simulink model "deadbeat_running_control"  (R2016b)
settings: configuration reference "Configuration1khz" (kept outside this file)
undefined symbols (not defined in the file or in its folder): A_kalman_no_position, A_kalman_transverse, A_kalman_vertical, A_lpf_accelerometer, A_lpf_contact, A_lpf_imu, A_lpf_lateral_angle, B1_lpf_accelerometer, B1_lpf_contact, B1_lpf_imu, B1_lpf_lateral_angle, B2_lpf_accelerometer, B2_lpf_contact, B2_lpf_imu, B2_lpf_lateral_angle, B_dx_versus_x0, B_kalman_no_position, B_kalman_transverse, B_kalman_vertical, backwards_K_sag_of_t, backwards_P_sag_of_t, C_kalman_no_position, C_kalman_transverse, C_kalman_vertical, com_leg_motor, com_torso, contact_threshold, d_ankle_to_foot, d_vertical_com, desired_com_forward_velocity, desired_com_lateral_velocity, desired_standing_torso_pitch, desired_standing_torso_roll, desired_standing_z, desired_torso_pitch, desired_torso_roll, DiscIntNeverNeededParam, Discrete, enable_bouncing, fdesignblkfcn, flight_duration, forward_dx_of_dxstar, forward_x_of_dxstar, g, gcbh, HIP_MTR_MAX_CONT_TORQUE, HIP_MTR_MAX_TORQUE, i_leg_motor, i_robot, i_torso, initial_dx_estimate, initial_dx_takeoff_history, initial_dx_touchdown_history, initial_dy_estimate, initial_dy_takeoff_history, initial_dy_touchdown_history, initial_dz_estimate, initial_leg_selection, initial_target_dx_history, initial_target_dy_history ... (+80)
libraries: simulink x22, ctrlSharedLib x4, dsparch4 x2
(part 3 of 7)

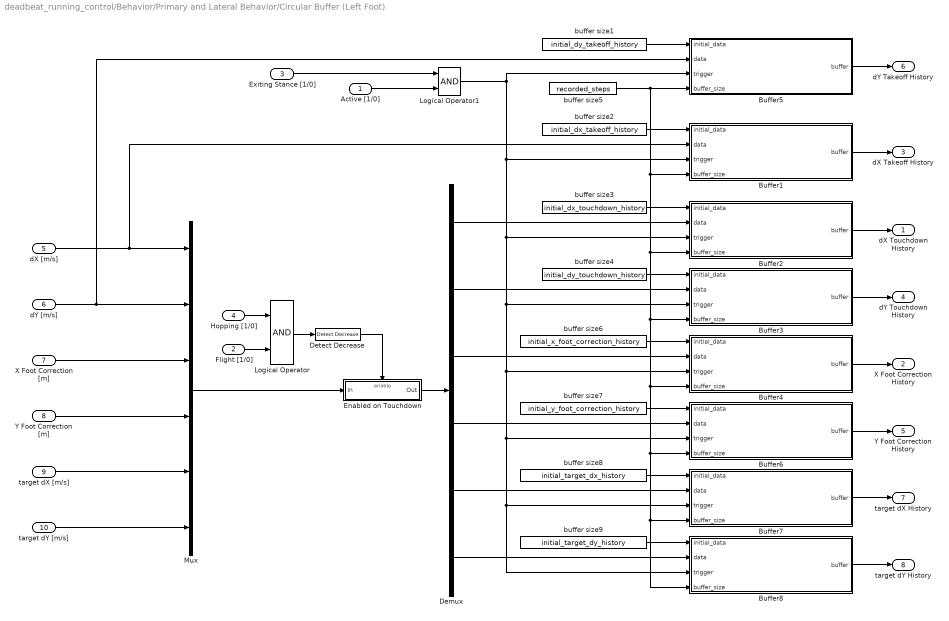
== system deadbeat_running_control/Behavior/Primary and Lateral Behavior/Circular Buffer (Left Foot) ==
  Active [1/0] : Inport
  Flight [1/0] : Inport  Port=2
  Exiting Stance [1/0] : Inport  Port=3
  Hopping [1/0] : Inport  Port=4
  dX [m/s] : Inport  Port=5
  dY [m/s] : Inport  Port=6
  X Foot Correction [m] : Inport  Port=7
  Y Foot Correction [m] : Inport  Port=8
  target dX [m/s] : Inport  Port=9
  target dY [m/s] : Inport  Port=10
  Buffer1 : MATLAB Function  TreatAsAtomicUnit=on  SystemSampleTime=sample_time
  Buffer2 : MATLAB Function  TreatAsAtomicUnit=on  SystemSampleTime=sample_time
  Buffer3 : MATLAB Function  TreatAsAtomicUnit=on  SystemSampleTime=sample_time
  Buffer4 : MATLAB Function  TreatAsAtomicUnit=on  SystemSampleTime=sample_time
  Buffer5 : MATLAB Function  TreatAsAtomicUnit=on  SystemSampleTime=sample_time
  Buffer6 : MATLAB Function  TreatAsAtomicUnit=on  SystemSampleTime=sample_time
  Buffer7 : MATLAB Function  TreatAsAtomicUnit=on  SystemSampleTime=sample_time
  Buffer8 : MATLAB Function  TreatAsAtomicUnit=on  SystemSampleTime=sample_time
  Demux : Demux  Outputs=6
  Detect Decrease : simulink/Logic and Bit Operations/Detect Decrease  vinit=0.0  InputProcessing=Inherited  OutDataTypeStr=boolean
  Enabled on Touchdown : Subsystem  TreatAsAtomicUnit=on
  Logical Operator : Logic  AllPortsSameDT=off  OutDataTypeStr=boolean
  Logical Operator1 : Logic  AllPortsSameDT=off  OutDataTypeStr=boolean
  Mux : Mux  Inputs=6
  buffer size1 : Constant  Value=initial_dy_takeoff_history
  buffer size2 : Constant  Value=initial_dx_takeoff_history
  buffer size3 : Constant  Value=initial_dx_touchdown_history
  buffer size4 : Constant  Value=initial_dy_touchdown_history
  buffer size5 : Constant  Value=recorded_steps
  buffer size6 : Constant  Value=initial_x_foot_correction_history
  buffer size7 : Constant  Value=initial_y_foot_correction_history
  buffer size8 : Constant  Value=initial_target_dx_history
  buffer size9 : Constant  Value=initial_target_dy_history
  "dX Touchdown History " : Outport
  X Foot Correction History : Outport  Port=2
  dX Takeoff History : Outport  Port=3
  "dY Touchdown History " : Outport  Port=4
  Y Foot Correction History : Outport  Port=5
  dY Takeoff History : Outport  Port=6
  target dX History : Outport  Port=7
  target dY History : Outport  Port=8
  wires:
  Enabled on Touchdown/1(Out) -> Demux/1
  Mux/1 -> Enabled on Touchdown/1(In)
  Logical Operator/1 -> Detect Decrease/1
  Flight [1/0]/1 -> Logical Operator/2
  dX [m/s]/1 -> Mux/1, Buffer1/2(data)
  dY [m/s]/1 -> Mux/2, Buffer5/2(data)
  Hopping [1/0]/1 -> Logical Operator/1
  Logical Operator1/1 -> Buffer7/3(trigger), Buffer8/3(trigger), Buffer6/3(trigger), Buffer4/3(trigger), Buffer3/3(trigger), Buffer2/3(trigger), Buffer1/3(trigger), Buffer5/3(trigger)
  target dY [m/s]/1 -> Mux/6
  Demux/5 -> Buffer7/2(data)
  Demux/6 -> Buffer8/2(data)
  buffer size5/1 -> Buffer5/4(buffer_size), Buffer7/4(buffer_size), Buffer8/4(buffer_size), Buffer6/4(buffer_size), Buffer4/4(buffer_size), Buffer3/4(buffer_size), Buffer2/4(buffer_size), Buffer1/4(buffer_size)
  Buffer8/1(buffer) -> target dY History/1
  Buffer7/1(buffer) -> target dX History/1
  target dX [m/s]/1 -> Mux/5
  Demux/4 -> Buffer6/2(data)
  Y Foot Correction [m]/1 -> Mux/4
  Buffer5/1(buffer) -> dY Takeoff History/1
  Demux/2 -> Buffer3/2(data)
  Buffer6/1(buffer) -> Y Foot Correction History/1
  Buffer3/1(buffer) -> "dY Touchdown History "/1
  X Foot Correction [m]/1 -> Mux/3
  Demux/3 -> Buffer4/2(data)
  Demux/1 -> Buffer2/2(data)
  Buffer1/1(buffer) -> dX Takeoff History/1
  Buffer4/1(buffer) -> X Foot Correction History/1
  Detect Decrease/1 -> Enabled on Touchdown/Enable
  Buffer2/1(buffer) -> "dX Touchdown History "/1
  buffer size1/1 -> Buffer5/1(initial_data)
  buffer size2/1 -> Buffer1/1(initial_data)
  buffer size3/1 -> Buffer2/1(initial_data)
  buffer size4/1 -> Buffer3/1(initial_data)
  buffer size6/1 -> Buffer4/1(initial_data)
  buffer size7/1 -> Buffer6/1(initial_data)
  buffer size8/1 -> Buffer7/1(initial_data)
  buffer size9/1 -> Buffer8/1(initial_data)
  Active [1/0]/1 -> Logical Operator1/2
  Exiting Stance [1/0]/1 -> Logical Operator1/1

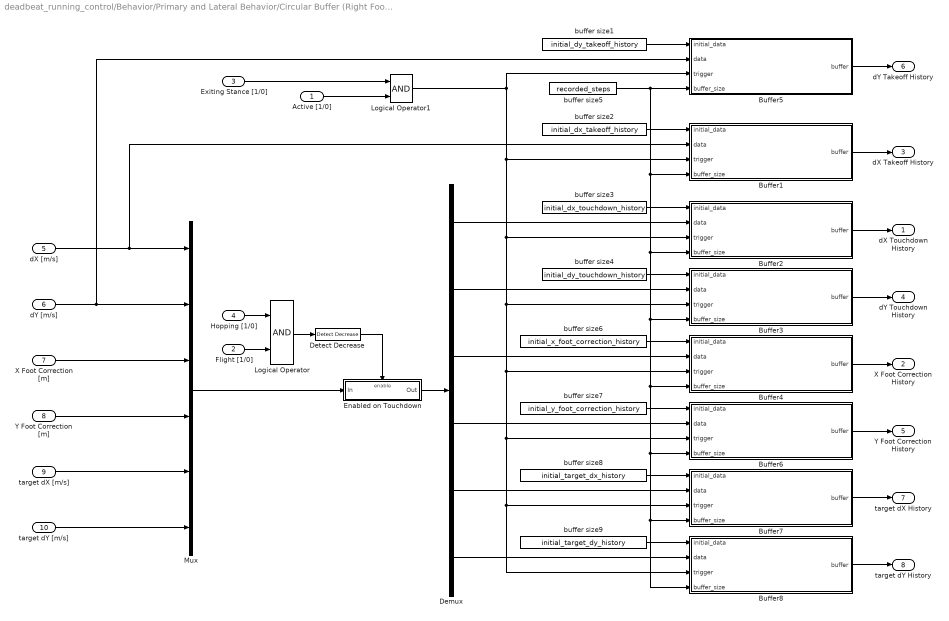
== system deadbeat_running_control/Behavior/Primary and Lateral Behavior/Circular Buffer (Right Foot) ==
  Active [1/0] : Inport
  Flight [1/0] : Inport  Port=2
  Exiting Stance [1/0] : Inport  Port=3
  Hopping [1/0] : Inport  Port=4
  dX [m/s] : Inport  Port=5
  dY [m/s] : Inport  Port=6
  X Foot Correction [m] : Inport  Port=7
  Y Foot Correction [m] : Inport  Port=8
  target dX [m/s] : Inport  Port=9
  target dY [m/s] : Inport  Port=10
  Buffer1 : MATLAB Function  TreatAsAtomicUnit=on  SystemSampleTime=sample_time
  Buffer2 : MATLAB Function  TreatAsAtomicUnit=on  SystemSampleTime=sample_time
  Buffer3 : MATLAB Function  TreatAsAtomicUnit=on  SystemSampleTime=sample_time
  Buffer4 : MATLAB Function  TreatAsAtomicUnit=on  SystemSampleTime=sample_time
  Buffer5 : MATLAB Function  TreatAsAtomicUnit=on  SystemSampleTime=sample_time
  Buffer6 : MATLAB Function  TreatAsAtomicUnit=on  SystemSampleTime=sample_time
  Buffer7 : MATLAB Function  TreatAsAtomicUnit=on  SystemSampleTime=sample_time
  Buffer8 : MATLAB Function  TreatAsAtomicUnit=on  SystemSampleTime=sample_time
  Demux : Demux  Outputs=6
  Detect Decrease : simulink/Logic and Bit Operations/Detect Decrease  vinit=0.0  InputProcessing=Inherited  OutDataTypeStr=boolean
  Enabled on Touchdown : Subsystem  TreatAsAtomicUnit=on
  Logical Operator : Logic  AllPortsSameDT=off  OutDataTypeStr=boolean
  Logical Operator1 : Logic  AllPortsSameDT=off  OutDataTypeStr=boolean
  Mux : Mux  Inputs=6
  buffer size1 : Constant  Value=initial_dy_takeoff_history
  buffer size2 : Constant  Value=initial_dx_takeoff_history
  buffer size3 : Constant  Value=initial_dx_touchdown_history
  buffer size4 : Constant  Value=initial_dy_touchdown_history
  buffer size5 : Constant  Value=recorded_steps
  buffer size6 : Constant  Value=initial_x_foot_correction_history
  buffer size7 : Constant  Value=initial_y_foot_correction_history
  buffer size8 : Constant  Value=initial_target_dx_history
  buffer size9 : Constant  Value=initial_target_dy_history
  "dX Touchdown History " : Outport
  X Foot Correction History : Outport  Port=2
  dX Takeoff History : Outport  Port=3
  "dY Touchdown History " : Outport  Port=4
  Y Foot Correction History : Outport  Port=5
  dY Takeoff History : Outport  Port=6
  target dX History : Outport  Port=7
  target dY History : Outport  Port=8
  wires:
  buffer size9/1 -> Buffer8/1(initial_data)
  buffer size8/1 -> Buffer7/1(initial_data)
  buffer size7/1 -> Buffer6/1(initial_data)
  buffer size6/1 -> Buffer4/1(initial_data)
  buffer size4/1 -> Buffer3/1(initial_data)
  buffer size3/1 -> Buffer2/1(initial_data)
  buffer size2/1 -> Buffer1/1(initial_data)
  buffer size1/1 -> Buffer5/1(initial_data)
  Buffer2/1(buffer) -> "dX Touchdown History "/1
  Detect Decrease/1 -> Enabled on Touchdown/Enable
  Buffer4/1(buffer) -> X Foot Correction History/1
  Buffer1/1(buffer) -> dX Takeoff History/1
  Demux/1 -> Buffer2/2(data)
  Demux/3 -> Buffer4/2(data)
  X Foot Correction [m]/1 -> Mux/3
  Buffer3/1(buffer) -> "dY Touchdown History "/1
  Buffer6/1(buffer) -> Y Foot Correction History/1
  Demux/2 -> Buffer3/2(data)
  Buffer5/1(buffer) -> dY Takeoff History/1
  Y Foot Correction [m]/1 -> Mux/4
  Demux/4 -> Buffer6/2(data)
  target dX [m/s]/1 -> Mux/5
  Buffer7/1(buffer) -> target dX History/1
  Buffer8/1(buffer) -> target dY History/1
  buffer size5/1 -> Buffer1/4(buffer_size), Buffer2/4(buffer_size), Buffer3/4(buffer_size), Buffer4/4(buffer_size), Buffer6/4(buffer_size), Buffer8/4(buffer_size), Buffer7/4(buffer_size), Buffer5/4(buffer_size)
  Demux/6 -> Buffer8/2(data)
  Demux/5 -> Buffer7/2(data)
  target dY [m/s]/1 -> Mux/6
  Logical Operator1/1 -> Buffer5/3(trigger), Buffer1/3(trigger), Buffer2/3(trigger), Buffer3/3(trigger), Buffer4/3(trigger), Buffer6/3(trigger), Buffer8/3(trigger), Buffer7/3(trigger)
  Hopping [1/0]/1 -> Logical Operator/1
  dY [m/s]/1 -> Buffer5/2(data), Mux/2
  dX [m/s]/1 -> Buffer1/2(data), Mux/1
  Flight [1/0]/1 -> Logical Operator/2
  Logical Operator/1 -> Detect Decrease/1
  Mux/1 -> Enabled on Touchdown/1(In)
  Enabled on Touchdown/1(Out) -> Demux/1
  Exiting Stance [1/0]/1 -> Logical Operator1/1
  Active [1/0]/1 -> Logical Operator1/2

== system deadbeat_running_control/Behavior/Primary and Lateral Behavior/Closed Loop Compensation (Left Foot) ==
  dX Touchdown History : Inport
  X Foot Correction History : Inport  Port=2
  dX Takeoff History : Inport  Port=3
  dY Touchdown History : Inport  Port=4
  Y Foot Correction History : Inport  Port=5
  dY Takeoff History : Inport  Port=6
  target dX History : Inport  Port=7
  target dY History : Inport  Port=8
  dX [m/s] : Inport  Port=9
  dY [m/s] : Inport  Port=10
  target dX [m/s] : Inport  Port=11
  "target dY [m/s] " : Inport  Port=12
  "A, eps, c" : Scope  NumInputPorts=3
  A_x_no_bias : Gain
  A_y_no_bias : Gain
  CLOSED LOOP COMPENSATION X FOR VAIRABLE SPEED : MATLAB Function  TreatAsAtomicUnit=on
  CLOSED LOOP COMPENSATION Y FOR VAIRABLE SPEED : MATLAB Function  TreatAsAtomicUnit=on
  Constant4 : Constant  Value=B_dx_versus_x0
  ESTIMATE CLOSED LOOP ERROR X FOR VARIABLE SPEED : MATLAB Function  TreatAsAtomicUnit=on
  ESTIMATE CLOSED LOOP ERROR Y FOR VARIABLE SPEED : MATLAB Function  TreatAsAtomicUnit=on
  How much dx depends on x0 : Constant  Value=B_dx_versus_x0
  RealVsFakeWeight : Constant  Value=2
  RealVsFakeWeight1 : Constant  Value=2
  Sum : Sum  Inputs=|+-
  Sum1 : Sum  Inputs=|+-
  Terminator{2..7} (6 alike) : Terminator
  XY Foot Correction : Scope  NumInputPorts=2
  c_x_no_bias : Gain
  c_y_no_bias : Gain
  epsilon_x_no_bias : Gain
  epsilon_y_no_bias : Gain
  X Foot Correction [m] : Outport
  Y Foot Correction [m] : Outport  Port=2
  wires:
  RealVsFakeWeight1/1 -> ESTIMATE CLOSED LOOP ERROR Y FOR VARIABLE SPEED/5(W_real)
  Constant4/1 -> CLOSED LOOP COMPENSATION Y FOR VAIRABLE SPEED/6(B_cl)
  "target dY [m/s] "/1 -> Sum1/2, CLOSED LOOP COMPENSATION Y FOR VAIRABLE SPEED/5(dx_star)
  target dY History/1 -> ESTIMATE CLOSED LOOP ERROR Y FOR VARIABLE SPEED/4(dx_star_hist)
  Y Foot Correction History/1 -> ESTIMATE CLOSED LOOP ERROR Y FOR VARIABLE SPEED/2(delta_ux_hist)
  dY Takeoff History/1 -> ESTIMATE CLOSED LOOP ERROR Y FOR VARIABLE SPEED/3(dx_lift_hist)
  dY [m/s]/1 -> Sum1/1
  RealVsFakeWeight/1 -> ESTIMATE CLOSED LOOP ERROR X FOR VARIABLE SPEED/5(W_real)
  How much dx depends on x0/1 -> CLOSED LOOP COMPENSATION X FOR VAIRABLE SPEED/6(B_cl)
  Sum/1 -> CLOSED LOOP COMPENSATION X FOR VAIRABLE SPEED/4(delta_s_i)
  target dX [m/s]/1 -> Sum/2, CLOSED LOOP COMPENSATION X FOR VAIRABLE SPEED/5(dx_star)
  target dX History/1 -> ESTIMATE CLOSED LOOP ERROR X FOR VARIABLE SPEED/4(dx_star_hist)
  X Foot Correction History/1 -> ESTIMATE CLOSED LOOP ERROR X FOR VARIABLE SPEED/2(delta_ux_hist)
  dX Takeoff History/1 -> ESTIMATE CLOSED LOOP ERROR X FOR VARIABLE SPEED/3(dx_lift_hist)
  dX Touchdown History/1 -> ESTIMATE CLOSED LOOP ERROR X FOR VARIABLE SPEED/1(dx_land_hist)
  dX [m/s]/1 -> Sum/1
  dY Touchdown History/1 -> ESTIMATE CLOSED LOOP ERROR Y FOR VARIABLE SPEED/1(dx_land_hist)
  Sum1/1 -> CLOSED LOOP COMPENSATION Y FOR VAIRABLE SPEED/4(delta_s_i)
  CLOSED LOOP COMPENSATION X FOR VAIRABLE SPEED/1(delta_ux) -> XY Foot Correction/1, X Foot Correction [m]/1
  CLOSED LOOP COMPENSATION Y FOR VAIRABLE SPEED/1(delta_ux) -> XY Foot Correction/2, Y Foot Correction [m]/1
  ESTIMATE CLOSED LOOP ERROR X FOR VARIABLE SPEED/6(c_nb) -> c_x_no_bias/1
  ESTIMATE CLOSED LOOP ERROR X FOR VARIABLE SPEED/5(epsilon_0_nb) -> epsilon_x_no_bias/1
  ESTIMATE CLOSED LOOP ERROR X FOR VARIABLE SPEED/4(A_cl_nb) -> A_x_no_bias/1
  A_x_no_bias/1 -> Terminator5/1
  epsilon_x_no_bias/1 -> Terminator6/1
  c_x_no_bias/1 -> Terminator7/1
  A_y_no_bias/1 -> Terminator2/1
  epsilon_y_no_bias/1 -> Terminator3/1
  c_y_no_bias/1 -> Terminator4/1
  ESTIMATE CLOSED LOOP ERROR Y FOR VARIABLE SPEED/4(A_cl_nb) -> A_y_no_bias/1
  ESTIMATE CLOSED LOOP ERROR Y FOR VARIABLE SPEED/5(epsilon_0_nb) -> epsilon_y_no_bias/1
  ESTIMATE CLOSED LOOP ERROR Y FOR VARIABLE SPEED/6(c_nb) -> c_y_no_bias/1
  ESTIMATE CLOSED LOOP ERROR X FOR VARIABLE SPEED/3(c) -> "A, eps, c"/3, CLOSED LOOP COMPENSATION X FOR VAIRABLE SPEED/3(c)
  ESTIMATE CLOSED LOOP ERROR X FOR VARIABLE SPEED/2(epsilon_0) -> "A, eps, c"/2, CLOSED LOOP COMPENSATION X FOR VAIRABLE SPEED/2(epsilon)
  ESTIMATE CLOSED LOOP ERROR X FOR VARIABLE SPEED/1(A_cl) -> CLOSED LOOP COMPENSATION X FOR VAIRABLE SPEED/1(A_cl), "A, eps, c"/1
  ESTIMATE CLOSED LOOP ERROR Y FOR VARIABLE SPEED/3(c) -> CLOSED LOOP COMPENSATION Y FOR VAIRABLE SPEED/3(c)
  ESTIMATE CLOSED LOOP ERROR Y FOR VARIABLE SPEED/2(epsilon_0) -> CLOSED LOOP COMPENSATION Y FOR VAIRABLE SPEED/2(epsilon)
  ESTIMATE CLOSED LOOP ERROR Y FOR VARIABLE SPEED/1(A_cl) -> CLOSED LOOP COMPENSATION Y FOR VAIRABLE SPEED/1(A_cl)

== system deadbeat_running_control/Behavior/Primary and Lateral Behavior/Closed Loop Compensation (Right Foot) ==
  dX Touchdown History : Inport
  X Foot Correction History : Inport  Port=2
  dX Takeoff History : Inport  Port=3
  dY Touchdown History : Inport  Port=4
  Y Foot Correction History : Inport  Port=5
  dY Takeoff History : Inport  Port=6
  target dX History : Inport  Port=7
  target dY History : Inport  Port=8
  dX [m/s] : Inport  Port=9
  dY [m/s] : Inport  Port=10
  target dX [m/s] : Inport  Port=11
  "target dY [m/s] " : Inport  Port=12
  "A, eps, c" : Scope  NumInputPorts=3
  A_x_no_bias : Gain
  A_y_no_bias : Gain
  CLOSED LOOP COMPENSATION X FOR VAIRABLE SPEED : MATLAB Function  TreatAsAtomicUnit=on
  CLOSED LOOP COMPENSATION Y FOR VAIRABLE SPEED : MATLAB Function  TreatAsAtomicUnit=on
  Constant4 : Constant  Value=B_dx_versus_x0
  ESTIMATE CLOSED LOOP ERROR X FOR VARIABLE SPEED : MATLAB Function  TreatAsAtomicUnit=on
  ESTIMATE CLOSED LOOP ERROR Y FOR VARIABLE SPEED : MATLAB Function  TreatAsAtomicUnit=on
  How much dx depends on x0 : Constant  Value=B_dx_versus_x0
  RealVsFakeWeight : Constant  Value=2
  RealVsFakeWeight1 : Constant  Value=2
  Sum : Sum  Inputs=|+-
  Sum1 : Sum  Inputs=|+-
  Terminator{2..7} (6 alike) : Terminator
  XY Foot Correction : Scope  NumInputPorts=2
  c_x_no_bias : Gain
  c_y_no_bias : Gain
  epsilon_x_no_bias : Gain
  epsilon_y_no_bias : Gain
  X Foot Correction [m] : Outport
  Y Foot Correction [m] : Outport  Port=2
  wires:
  ESTIMATE CLOSED LOOP ERROR Y FOR VARIABLE SPEED/1(A_cl) -> CLOSED LOOP COMPENSATION Y FOR VAIRABLE SPEED/1(A_cl)
  ESTIMATE CLOSED LOOP ERROR Y FOR VARIABLE SPEED/2(epsilon_0) -> CLOSED LOOP COMPENSATION Y FOR VAIRABLE SPEED/2(epsilon)
  ESTIMATE CLOSED LOOP ERROR Y FOR VARIABLE SPEED/3(c) -> CLOSED LOOP COMPENSATION Y FOR VAIRABLE SPEED/3(c)
  ESTIMATE CLOSED LOOP ERROR X FOR VARIABLE SPEED/1(A_cl) -> "A, eps, c"/1, CLOSED LOOP COMPENSATION X FOR VAIRABLE SPEED/1(A_cl)
  ESTIMATE CLOSED LOOP ERROR X FOR VARIABLE SPEED/2(epsilon_0) -> CLOSED LOOP COMPENSATION X FOR VAIRABLE SPEED/2(epsilon), "A, eps, c"/2
  ESTIMATE CLOSED LOOP ERROR X FOR VARIABLE SPEED/3(c) -> CLOSED LOOP COMPENSATION X FOR VAIRABLE SPEED/3(c), "A, eps, c"/3
  ESTIMATE CLOSED LOOP ERROR Y FOR VARIABLE SPEED/6(c_nb) -> c_y_no_bias/1
  ESTIMATE CLOSED LOOP ERROR Y FOR VARIABLE SPEED/5(epsilon_0_nb) -> epsilon_y_no_bias/1
  ESTIMATE CLOSED LOOP ERROR Y FOR VARIABLE SPEED/4(A_cl_nb) -> A_y_no_bias/1
  c_y_no_bias/1 -> Terminator4/1
  epsilon_y_no_bias/1 -> Terminator3/1
  A_y_no_bias/1 -> Terminator2/1
  c_x_no_bias/1 -> Terminator7/1
  epsilon_x_no_bias/1 -> Terminator6/1
  A_x_no_bias/1 -> Terminator5/1
  ESTIMATE CLOSED LOOP ERROR X FOR VARIABLE SPEED/4(A_cl_nb) -> A_x_no_bias/1
  ESTIMATE CLOSED LOOP ERROR X FOR VARIABLE SPEED/5(epsilon_0_nb) -> epsilon_x_no_bias/1
  ESTIMATE CLOSED LOOP ERROR X FOR VARIABLE SPEED/6(c_nb) -> c_x_no_bias/1
  CLOSED LOOP COMPENSATION Y FOR VAIRABLE SPEED/1(delta_ux) -> Y Foot Correction [m]/1, XY Foot Correction/2
  CLOSED LOOP COMPENSATION X FOR VAIRABLE SPEED/1(delta_ux) -> X Foot Correction [m]/1, XY Foot Correction/1
  Sum1/1 -> CLOSED LOOP COMPENSATION Y FOR VAIRABLE SPEED/4(delta_s_i)
  dY Touchdown History/1 -> ESTIMATE CLOSED LOOP ERROR Y FOR VARIABLE SPEED/1(dx_land_hist)
  dX [m/s]/1 -> Sum/1
  dX Touchdown History/1 -> ESTIMATE CLOSED LOOP ERROR X FOR VARIABLE SPEED/1(dx_land_hist)
  dX Takeoff History/1 -> ESTIMATE CLOSED LOOP ERROR X FOR VARIABLE SPEED/3(dx_lift_hist)
  X Foot Correction History/1 -> ESTIMATE CLOSED LOOP ERROR X FOR VARIABLE SPEED/2(delta_ux_hist)
  target dX History/1 -> ESTIMATE CLOSED LOOP ERROR X FOR VARIABLE SPEED/4(dx_star_hist)
  target dX [m/s]/1 -> CLOSED LOOP COMPENSATION X FOR VAIRABLE SPEED/5(dx_star), Sum/2
  Sum/1 -> CLOSED LOOP COMPENSATION X FOR VAIRABLE SPEED/4(delta_s_i)
  How much dx depends on x0/1 -> CLOSED LOOP COMPENSATION X FOR VAIRABLE SPEED/6(B_cl)
  RealVsFakeWeight/1 -> ESTIMATE CLOSED LOOP ERROR X FOR VARIABLE SPEED/5(W_real)
  dY [m/s]/1 -> Sum1/1
  dY Takeoff History/1 -> ESTIMATE CLOSED LOOP ERROR Y FOR VARIABLE SPEED/3(dx_lift_hist)
  Y Foot Correction History/1 -> ESTIMATE CLOSED LOOP ERROR Y FOR VARIABLE SPEED/2(delta_ux_hist)
  target dY History/1 -> ESTIMATE CLOSED LOOP ERROR Y FOR VARIABLE SPEED/4(dx_star_hist)
  "target dY [m/s] "/1 -> CLOSED LOOP COMPENSATION Y FOR VAIRABLE SPEED/5(dx_star), Sum1/2
  Constant4/1 -> CLOSED LOOP COMPENSATION Y FOR VAIRABLE SPEED/6(B_cl)
  RealVsFakeWeight1/1 -> ESTIMATE CLOSED LOOP ERROR Y FOR VARIABLE SPEED/5(W_real)

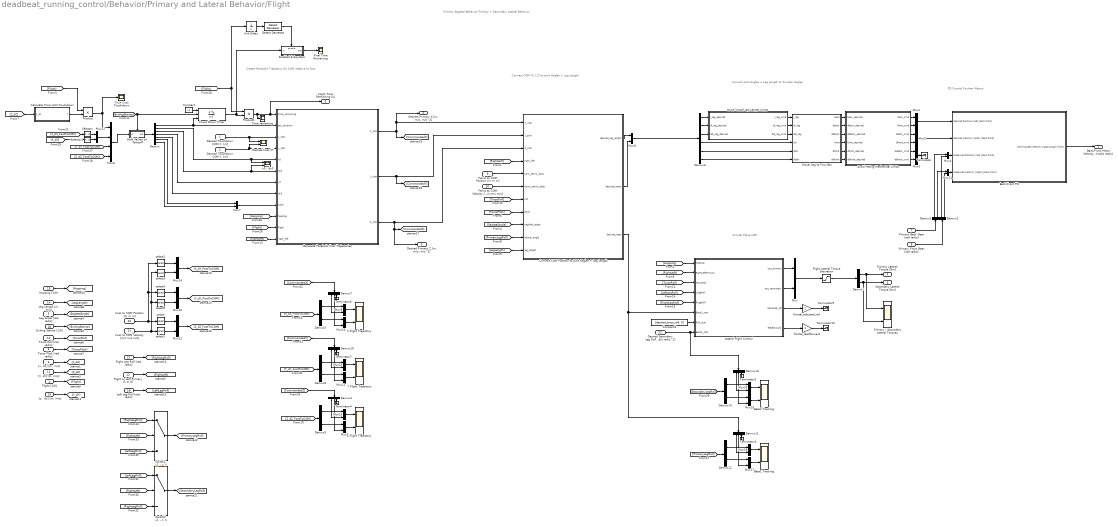
== system deadbeat_running_control/Behavior/Primary and Lateral Behavior/Flight ==
  note: Frontal Plane LQR
  note: PD Control Fourbar Motors
  note: Convert Joint Angles + Leg Length
      | to Fourbar Angles
  note: Convert COM (X,Y,Z) to
      | Joint Angles + Leg Length
  note: Create Parabolic
      | Trajectory for COM relative to foot
  note: Primary Sagittal Behavior
      | Primary + Secondary Lateral Behavior
  Desired Touchdown COM X  [m] : Inport
  Desired Touchdown COM Y  [m] : Inport  Port=2
  Torso Pitch [rad rad/s] : Inport  Port=3
  Flight [1/0] : Inport  Port=4
  Leg Angle [rad rad/s] : Inport  Port=5
  "[x, dx] [m, m/s]" : Inport  Port=6
  Primary Back Gear [rad rad/s] : Inport  Port=7
  Primary Front Gear [rad rad/s] : Inport  Port=8
  Pelvis to COM Position [m m m] : Inport  Port=9
  Pelvis to COM Velocity [m/s m/s m/s] : Inport  Port=10
  "[z, dz] [m, m/s]" : Inport  Port=11
  Right or Left Primary [1 or 0] : Inport  Port=12
  Torso Roll [rad rad/s] : Inport  Port=13
  "Leg Length [m, m/s]" : Inport  Port=14
  "[y,  dy] [m, m/s]" : Inport  Port=15
  "Left Leg Roll [rad, rad/s]" : Inport  Port=16
  "Right Leg Roll [rad, rad/s]" : Inport  Port=17
  Exiting Stance [1/0] : Inport  Port=18
  Hopping [1/0] : Inport  Port=19
  Foot to COM Position [m m m] : Inport  Port=20
  Foot to COM Velocity [m/s m/s m/s] : Inport  Port=21
  Desired Secondary Leg Roll [rad rad/s rad/s^2] : Inport  Port=22
  Avoid Hitting Mechanical Limits : MATLAB Function  TreatAsAtomicUnit=on
  Avoid Virtual Leg Length Limits : MATLAB Function  TreatAsAtomicUnit=on
  Back/Front PD : Subsystem
  Beta1 Tracking : Scope  NumInputPorts=2
  Beta2 Tracking : Scope  NumInputPorts=2
  Calculate Time Until Touchdown : MATLAB Function  TreatAsAtomicUnit=on
  Constant : Constant  Value=-1
  Constant1 : Constant  Value=[desired_torso_roll; 0]
  "Convert COM Position to Joint Angles + Leg Length " : MATLAB Function  TreatAsAtomicUnit=on
  Count Down Timer : DiscreteIntegrator  ExternalReset=rising  InitialConditionSource=external  InitialConditionSetting=State (most efficient)  SampleTime=sample_time  LimitOutput=on  LowerSaturationLimit=0  ICPrevOutput=DiscIntNeverNeededParam  ICPrevScaledInput=DiscIntNeverNeededParam
  Demux : Demux  Outputs=7
  Demux{1..3,5,8..9,12,14} (8 alike) : Demux  Outputs=2
  Demux{4,7,10..11,13} (5 alike) : Demux  Outputs=3
  Demux6 : Demux  Outputs=6
  Desired Foot XY : Scope  NumInputPorts=2
  Detect Decrease : simulink/Logic and Bit Operations/Detect Decrease  vinit=0.0  InputProcessing=Inherited  OutDataTypeStr=boolean
  Enabled Subsystem : Subsystem  TreatAsAtomicUnit=on
  Final Time Remaining : Scope
  Flight Lateral Torque Saturation : Saturate  UpperLimit=HIP_MTR_MAX_CONT_TORQUE  LowerLimit=-HIP_MTR_MAX_CONT_TORQUE
      settings: AttributesFormatString=Top: %<UpperLimit>\nBottom: %<LowerLimit>
  Generate Parabolic Foot Trajectories : MATLAB Function  TreatAsAtomicUnit=on
  Hold Values on Takeoff : Subsystem
  Lateral Flight Control : MATLAB Function  TreatAsAtomicUnit=on
  Mux{,1..5,7..22} (22 alike) : Mux  Inputs=2
  Mux6 : Mux
  Primary / Secondary Lateral Torques : Scope  NumInputPorts=2
  Product : Product
  Product1 : Product
  Selector : Selector  InputPortWidth=2  IndexOptions=Index vector (dialog)  Indices=[1]  OutputSizes=1
  Selector1 : Selector  InputPortWidth=2  IndexOptions=Index vector (dialog)  Indices=[2]  OutputSizes=1
  Switch1 : Switch  Criteria=u2 ~= 0
  Switch2 : Switch  Criteria=u2 ~= 0
  Terminator{,1..2,4,6..7,9..10} (8 alike) : Terminator
  Time Until Touchdown : Scope
  Time remaining : Scope
  Unit Delay : UnitDelay  SampleTime=-1
  Virtual Leg to Four Bar : MATLAB Function  TreatAsAtomicUnit=on
  X Flight Trajectory : Scope  NumInputPorts=2
  Y Flight Trajectory : Scope  NumInputPorts=2
  Z Flight Trajectory : Scope  NumInputPorts=2
  frontal_adjusted_ref : Gain
  frontal_feedforward : Gain
  select : Selector  InputPortWidth=3  IndexOptions=Index vector (dialog)  Indices=[3]  OutputSizes=1
  select1 : Selector  InputPortWidth=3  IndexOptions=Index vector (dialog)  Indices=[3]  OutputSizes=1
  select2 : Selector  InputPortWidth=3  IndexOptions=Index vector (dialog)  Indices=[1]  OutputSizes=1
  select3 : Selector  InputPortWidth=3  IndexOptions=Index vector (dialog)  Indices=[1]  OutputSizes=1
  select4 : Selector  InputPortWidth=3  IndexOptions=Index vector (dialog)  Indices=[2]  OutputSizes=1
  select5 : Selector  InputPortWidth=3  IndexOptions=Index vector (dialog)  Indices=[2]  OutputSizes=1
  x0 / dx0 : Scope  NumInputPorts=2
  Back/Front Motor Velocity [rad/s rad/s] : Outport
  Primary Lateral Torque [Nm] : Outport  Port=2
  Secondary Lateral Torque [Nm] : Outport  Port=3
  "Desired Primary X [m, m/s, m/s^2]" : Outport  Port=4
  "Desired Primary Z [m, m/s, m/s^2]" : Outport  Port=5
  Flight Time Remaining [s] : Outport  Port=6
  wires:
  Desired Secondary Leg Roll [rad rad/s rad/s^2]/1 -> Demux13/1, Lateral Flight Control/8(Beta2_star)
  "Convert COM Position to Joint Angles + Leg Length "/3(desired_beta) -> Lateral Flight Control/6(Beta1_star), Demux11/1
  Demux11/3 -> Terminator1/1
  [PrimaryLegRoll] -> Demux12/1
  Demux11/2 -> Mux17/2
  Demux11/1 -> Mux18/2
  Demux12/2 -> Mux17/1
  Demux12/1 -> Mux18/1
  Mux17/1 -> Beta1 Tracking/2
  Mux18/1 -> Beta1 Tracking/1
  Unit Delay/1 -> Detect Decrease/1
  Detect Decrease/1 -> Enabled Subsystem/Enable
  Enabled Subsystem/1(out) -> Final Time Remaining/1
  [Flight] -> Product1/1, Unit Delay/1
  Product1/1 -> Flight Time Remaining [s]/1, Generate Parabolic Foot Trajectories/1(time_remaining), Time remaining/1
  Count Down Timer/1 -> Product1/2, Enabled Subsystem/1(in)
  Constant/1 -> Count Down Timer/1
  [Flight] -> Product/1
  Calculate Time Until Touchdown/1(t) -> Product/2
  Mux16/1 -> [Y_dY_FootToCOM]
  select5/1 -> Mux16/2
  select4/1 -> Mux16/1
  Foot to COM Velocity [m/s m/s m/s]/1 -> select1/1, select3/1, select5/1
  Foot to COM Position [m m m]/1 -> select/1, select2/1, select4/1
  Mux14/1 -> [X_dX_FootToCOM]
  select3/1 -> Mux14/2
  select2/1 -> Mux14/1
  Mux3/1 -> Terminator/1
  [CommandedZ] -> Demux4/1
  [CommandedY] -> Demux10/1
  [CommandedX] -> Demux7/1
  Demux10/3 -> Terminator7/1
  [Y_dY_FootToCOM] -> Demux8/1
  Demux10/2 -> Mux12/2
  Demux10/1 -> Mux13/2
  Demux8/2 -> Mux12/1
  Demux8/1 -> Mux13/1
  Mux12/1 -> Y Flight Trajectory/2
  Mux13/1 -> Y Flight Trajectory/1
  Demux7/3 -> Terminator6/1
  [X_dX_FootToCOM] -> Demux5/1
  Demux7/2 -> Mux10/2
  Demux7/1 -> Mux9/2
  Demux5/2 -> Mux10/1
  Demux5/1 -> Mux9/1
  Mux10/1 -> X Flight Trajectory/2
  Mux9/1 -> X Flight Trajectory/1
  Demux4/3 -> Terminator4/1
  Demux4/2 -> Mux5/2
  Demux4/1 -> Mux15/2
  Demux9/2 -> Mux5/1
  Demux9/1 -> Mux15/1
  [Z_dZ_FootToCOM] -> Demux9/1
  [Z_dZ_FootToCOM] -> Mux6/4
  Mux5/1 -> Z Flight Trajectory/2
  Mux15/1 -> Z Flight Trajectory/1
  Mux21/1 -> [Z_dZ_FootToCOM]
  select1/1 -> Mux21/2
  select/1 -> Mux21/1
  Demux/7 -> Mux7/2
  Demux/6 -> Mux7/1
  Demux/5 -> Generate Parabolic Foot Trajectories/8(dy0)
  Demux/4 -> Generate Parabolic Foot Trajectories/7(y0)
  Demux/3 -> x0 / dx0/2, Generate Parabolic Foot Trajectories/6(dx0)
  [Flight] -> Generate Parabolic Foot Trajectories/11(flight)
  Hopping [1/0]/1 -> [Hopping]
  [Hopping] -> Lateral Flight Control/1(hopping)
  Mux/1 -> Flight Lateral Torque Saturation/1
  frontal_adjusted_ref/1 -> Terminator9/1
  frontal_feedforward/1 -> Terminator10/1
  Flight Lateral Torque Saturation/1 -> Demux1/1
  Demux1/2 -> Secondary Lateral Torque [Nm]/1, Primary / Secondary Lateral Torques/2
  Demux1/1 -> Primary Lateral Torque [Nm]/1, Primary / Secondary Lateral Torques/1
  Exiting Stance [1/0]/1 -> [ExitingStance]
  Switch1/1 -> [PrimaryLegRoll]
  Right or Left Primary [1 or 0]/1 -> [RightLeft]
  "Right Leg Roll [rad, rad/s]"/1 -> [RightLegRoll]
  [RightLegRoll] -> Lateral Flight Control/5(RLegRoll)
  [LeftLegRoll] -> Lateral Flight Control/4(LLegRoll)
  "Left Leg Roll [rad, rad/s]"/1 -> [LeftLegRoll]
  Lateral Flight Control/1(tau_primary) -> Mux/1
  Lateral Flight Control/2(tau_secondary) -> Mux/2
  Lateral Flight Control/4(feedforward) -> frontal_feedforward/1
  Lateral Flight Control/3(adjusted_ref) -> frontal_adjusted_ref/1
  Constant1/1 -> Lateral Flight Control/7(Roll_star)
  [TorsoRoll] -> Lateral Flight Control/3(TorsoRoll)
  [RightLeft] -> Lateral Flight Control/2(RightLeftPrimary)
  Desired Touchdown COM Y  [m]/1 -> Desired Foot XY/2, Generate Parabolic Foot Trajectories/4(y_star)
  Demux6/3 -> Avoid Virtual Leg Length Limits/3(ddl_leg_desired)
  Demux6/2 -> Avoid Virtual Leg Length Limits/2(dl_leg_desired)
  Demux6/1 -> Avoid Virtual Leg Length Limits/1(l_leg_desired)
  Avoid Virtual Leg Length Limits/3(ddl_leg_cmd) -> Virtual Leg to Four Bar/3(ddl_leg)
  Avoid Virtual Leg Length Limits/2(dl_leg_cmd) -> Virtual Leg to Four Bar/2(dl_leg)
  Avoid Virtual Leg Length Limits/1(l_leg_cmd) -> Virtual Leg to Four Bar/1(l_leg)
  Product/1 -> Mux6/1, Time Until Touchdown/1
  [Z_dZ] -> Calculate Time Until Touchdown/1(z_dz)
  [Y_dY_FootToCOM] -> Mux6/3
  "[y,  dy] [m, m/s]"/1 -> [Y_dY]
  Desired Touchdown COM X  [m]/1 -> Generate Parabolic Foot Trajectories/3(x_star), Desired Foot XY/1
  "[z, dz] [m, m/s]"/1 -> [Z_dZ]
  "Leg Length [m, m/s]"/1 -> [LegLength]
  Torso Roll [rad rad/s]/1 -> [TorsoRoll]
  "[x, dx] [m, m/s]"/1 -> [X_dX]
  [ExitingStance] -> Count Down Timer/2, Hold Values on Takeoff/Trigger
  Flight [1/0]/1 -> [Flight]
  Pelvis to COM Velocity [m/s m/s m/s]/1 -> "Convert COM Position to Joint Angles + Leg Length "/6(dcom_pelvis_body)
  Pelvis to COM Position [m m m]/1 -> "Convert COM Position to Joint Angles + Leg Length "/5(com_pelvis_body)
  [TorsoRoll] -> "Convert COM Position to Joint Angles + Leg Length "/7(roll)
  [LegLength] -> "Convert COM Position to Joint Angles + Leg Length "/11(leg_length)
  [PrimaryLegRoll] -> "Convert COM Position to Joint Angles + Leg Length "/10(lateral_angle)
  [TorsoPitch] -> "Convert COM Position to Joint Angles + Leg Length "/8(pitch)
  Torso Pitch [rad rad/s]/1 -> [TorsoPitch]
  [SagittalAngle] -> "Convert COM Position to Joint Angles + Leg Length "/9(sagittal_angle)
  Leg Angle [rad rad/s]/1 -> [SagittalAngle]
  Mux8/1 -> Demux6/1
  Demux6/4 -> Virtual Leg to Four Bar/4(phi)
  Demux6/5 -> Virtual Leg to Four Bar/5(dphi)
  Demux6/6 -> Virtual Leg to Four Bar/6(ddphi)
  "Convert COM Position to Joint Angles + Leg Length "/1(desired_leg_length) -> Mux8/1
  "Convert COM Position to Joint Angles + Leg Length "/2(desired_alpha) -> Mux8/2
  [RightLeft] -> "Convert COM Position to Joint Angles + Leg Length "/4(right_left)
  Generate Parabolic Foot Trajectories/2(Y_star) -> [CommandedY], "Convert COM Position to Joint Angles + Leg Length "/2(Y_star)
  Generate Parabolic Foot Trajectories/1(X_star) -> "Desired Primary X [m, m/s, m/s^2]"/1, "Convert COM Position to Joint Angles + Leg Length "/1(X_star), [CommandedX]
  Mux22/1 -> Mux6/2
  Hold Values on Takeoff/1(out) -> Demux/1
  Mux6/1 -> Hold Values on Takeoff/1(in)
  Mux7/1 -> Generate Parabolic Foot Trajectories/9(zdz0)
  Demux/1 -> Generate Parabolic Foot Trajectories/2(est_duration), Count Down Timer/3
  Primary Front Gear [rad rad/s]/1 -> Demux2/1
  Primary Back Gear [rad rad/s]/1 -> Demux3/1
  Back/Front PD/1(Commanded Velocity [rad/s] [back front]) -> Back/Front Motor Velocity [rad/s rad/s]/1
  Mux2/1 -> Back/Front PD/2(Desired Velocity [rad/s] [back front])
  Avoid Hitting Mechanical Limits/6(ddfront_cmd) -> Mux3/2
  Avoid Hitting Mechanical Limits/5(ddback_cmd) -> Mux3/1
  Avoid Hitting Mechanical Limits/4(dfront_cmd) -> Mux2/2
  Avoid Hitting Mechanical Limits/3(dback_cmd) -> Mux2/1
  Demux2/1 -> Mux4/2
  Avoid Hitting Mechanical Limits/1(back_cmd) -> Mux1/1
  Avoid Hitting Mechanical Limits/2(front_cmd) -> Mux1/2
  Demux3/1 -> Mux4/1
  Demux3/2 -> Mux11/1
  Mux1/1 -> Back/Front PD/1(Desired Position [rad] [back front])
  Mux4/1 -> Back/Front PD/3(Measured Position [rad] [back front])
  Demux2/2 -> Mux11/2
  Mux11/1 -> Back/Front PD/4(Measured Velocity [rad/s] [back front])
  Virtual Leg to Four Bar/6(ddfront) -> Avoid Hitting Mechanical Limits/6(ddfront_desired)
  Virtual Leg to Four Bar/5(dfront) -> Avoid Hitting Mechanical Limits/5(dfront_desired)
  Virtual Leg to Four Bar/4(front) -> Avoid Hitting Mechanical Limits/4(front_desired)
  Virtual Leg to Four Bar/3(ddback) -> Avoid Hitting Mechanical Limits/3(ddback_desired)
  Virtual Leg to Four Bar/2(dback) -> Avoid Hitting Mechanical Limits/2(dback_desired)
  Virtual Leg to Four Bar/1(back) -> Avoid Hitting Mechanical Limits/1(back_desired)
  [RightLeft] -> Generate Parabolic Foot Trajectories/12(right_left)
  Demux13/3 -> Terminator2/1
  [SecondaryLegRoll] -> Demux14/1
  Demux13/2 -> Mux19/2
  Demux13/1 -> Mux20/2
  Demux14/2 -> Mux19/1
  Demux14/1 -> Mux20/1
  Mux19/1 -> Beta2 Tracking/2
  Mux20/1 -> Beta2 Tracking/1
  Switch2/1 -> [SecondaryLegRoll]
  [RightLeft] -> Switch2/2
  [LeftLegRoll] -> Switch2/1
  [RightLegRoll] -> Switch2/3
  [LeftLegRoll] -> Switch1/3
  [RightLeft] -> Switch1/2
  [RightLegRoll] -> Switch1/1
  Generate Parabolic Foot Trajectories/3(Z_star) -> "Desired Primary Z [m, m/s, m/s^2]"/1, [CommandedZ], "Convert COM Position to Joint Angles + Leg Length "/3(Z_star)
  [Hopping] -> Generate Parabolic Foot Trajectories/10(hopping)
  [X_dX_FootToCOM] -> Selector/1
  [X_dX] -> Selector1/1
  Selector/1 -> Mux22/1
  Selector1/1 -> Mux22/2
  Demux/2 -> x0 / dx0/1, Generate Parabolic Foot Trajectories/5(x0)

== system deadbeat_running_control/Behavior/Primary and Lateral Behavior/Hold Values on Takeoff ==
  in : Inport
  Trigger : TriggerPort  VariantControl=Variant  ShowOutputPort=on  PortDimensions=1
  Subsystem : Subsystem
  out : Outport
  wires:
  Trigger/1 -> Subsystem/Enable
  Subsystem/1(out) -> out/1
  in/1 -> Subsystem/1(in)

== system deadbeat_running_control/Behavior/Primary and Lateral Behavior/Hold Values on Takeoff1 ==
  in : Inport
  Trigger : TriggerPort  VariantControl=Variant  ShowOutputPort=on  PortDimensions=1
  Subsystem : Subsystem
  out : Outport
  wires:
  in/1 -> Subsystem/1(in)
  Subsystem/1(out) -> out/1
  Trigger/1 -> Subsystem/Enable

== system deadbeat_running_control/Behavior/Primary and Lateral Behavior/Hold Values on Takeoff2 ==
  in : Inport
  Trigger : TriggerPort  VariantControl=Variant  ShowOutputPort=on  PortDimensions=1
  Subsystem : Subsystem
  out : Outport
  wires:
  in/1 -> Subsystem/1(in)
  Subsystem/1(out) -> out/1
  Trigger/1 -> Subsystem/Enable

== system deadbeat_running_control/Behavior/Primary and Lateral Behavior/Hold Values on Takeoff3 ==
  in : Inport
  Trigger : TriggerPort  VariantControl=Variant  ShowOutputPort=on  PortDimensions=1
  Subsystem : Subsystem
  out : Outport
  wires:
  Trigger/1 -> Subsystem/Enable
  Subsystem/1(out) -> out/1
  in/1 -> Subsystem/1(in)
